simulink model "ps9_prob3_b_model"  (R2014a)
settings: Solver=ode45  StartTime=0.0  StopTime=10.0  RelTol=1e-3
values from neighbouring files (symbols this model uses):
  a_tf = a_temp    [compute_h_infty.m]
  w_0 = w_0_temp    [compute_h_infty.m]
settings Model: Creator=HP  LastModifiedBy=manuelli
settings DataIOCC: SignalLoggingSaveFormat=ModelDataLogs
settings OptimizationCC: ExpressionDepthLimit=2147483647
settings DebuggingCC: UnderspecifiedInitializationDetection=Classic  FcnCallInpInsideContextMsg=EnableAllAsWarning  StateNameClashWarn=warning

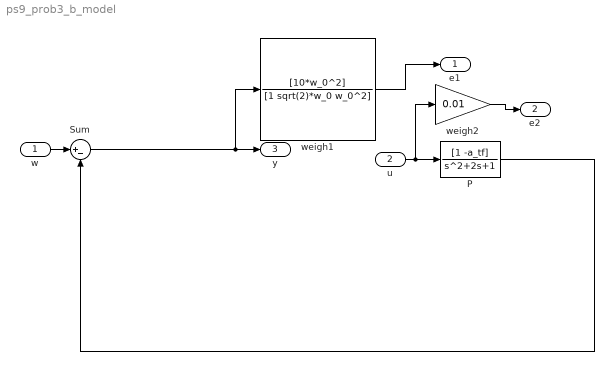
== system ps9_prob3_b_model ==
  w : Inport
  u : Inport  Port=2
  P : TransferFcn  Numerator=[1 -a_tf]
  Sum : Sum  Inputs=|+-
  weigh1 : TransferFcn  Numerator=[10*w_0^2]  Denominator=[1 sqrt(2)*w_0 w_0^2]
  weigh2 : Gain  Gain=0.01
  e1 : Outport
  e2 : Outport  Port=2
  y : Outport  Port=3
  wires:
  u/1 -> P/1, weigh2/1
  weigh1/1 -> e1/1
  w/1 -> Sum/1
  P/1 -> Sum/2
  weigh2/1 -> e2/1
  Sum/1 -> y/1, weigh1/1
